simulink model "GMSK_IO_modulator"  (R2024a)
settings: Solver=FixedStepAuto  StartTime=0.0  StopTime=10.0  FixedStep=DESIGN_CONST.Tsim  RelTol=1e-3
undefined symbols (not defined in the file or in its folder): DESIGN_CONST
settings Model: Creator=Sayantan  LastModifiedBy=Sayantan

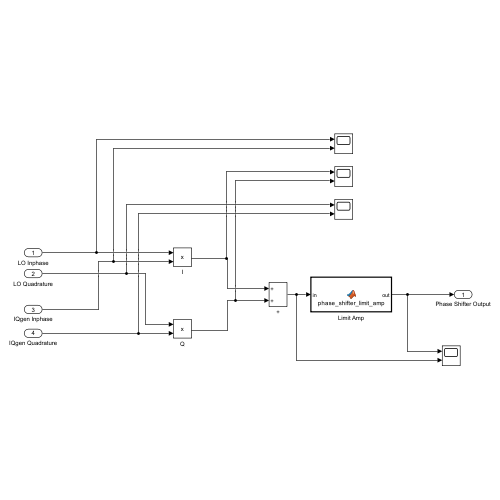
[thumbnail: Simulink's stored preview of the top-level diagram]
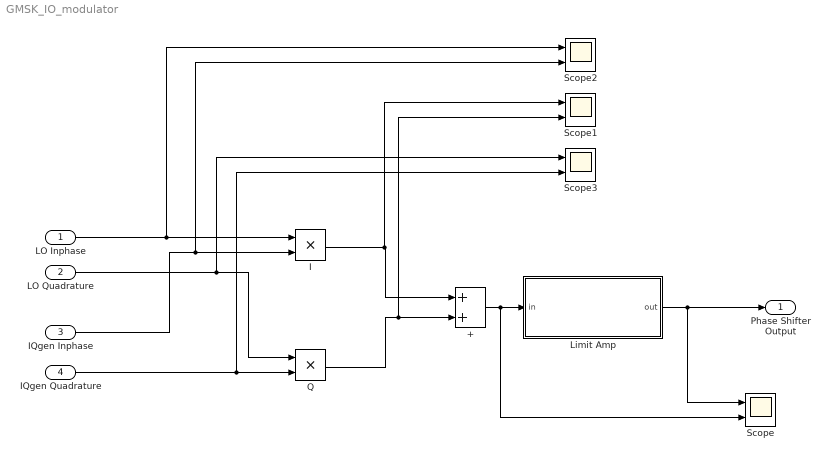
== system GMSK_IO_modulator ==
  LO Inphase : Inport
  LO Quadrature : Inport  Port=2
  IQgen Inphase : Inport  Port=3
  IQgen Quadrature : Inport  Port=4
  + : Sum  OutDataTypeStr=double
  I : Product
  Limit Amp : MATLAB Function  TreatAsAtomicUnit=on  SystemSampleTime=DESIGN_CONST.Tsim
  Q : Product
  Scope{,1..3} (4 alike) : Scope  NumInputPorts=2
  Phase Shifter Output : Outport
  wires:
  I/1 -> Scope1/1, +/1
  Q/1 -> Scope1/2, +/2
  +/1 -> Limit Amp/1(in), Scope/2
  LO Inphase/1 -> Scope2/1, I/1
  LO Quadrature/1 -> Scope3/1, Q/1
  IQgen Inphase/1 -> Scope2/2, I/2
  IQgen Quadrature/1 -> Scope3/2, Q/2
  Limit Amp/1(out) -> Scope/1, Phase Shifter Output/1

== matlab function GMSK_IO_modulator/Limit Amp ==
  data: in input; out output
function out  = phase_shifter_limit_amp(in)
%#codegen

% Persistent variables for state and previous input
persistent prev_in state val;

% Initialize persistent variables on the first call
if isempty(state)
    state = -2;
end
if isempty(prev_in)
    prev_in = 0.0;
end
if isempty(val)
    val = -1.0;
end

% Phase shifter and limit amplifier logic
if (state == -2 && in >= 0.0) % Positive transition
    val = (in + prev_in) / (in - prev_in);
    state = 1;
elseif (state == 1)
    val = 1.0;
    state = 2;
elseif (state == 2 && in < 0.0) % Negative transition
    val = -(in + prev_in) / (in - prev_in);
    state = -1;
elseif (state == -1)
    val = -1.0;
    state = -2;
end

% Update the previous input
out = val;

end
